simulink model "controle_manual_tuned_PID"  (Simulink 8.3)
settings: Solver=ode3  StartTime=0.0  StopTime=20  FixedStep=0.01  MaxStep=0.1  RelTol=1e-3
InitFcn:
  | % load parameters of the default quadrotor
  | disp('Quadrotor parameters loaded by InitFcn')
  | mdl_quadrotor
  | 
  | P_x=0.1;
  | I_x=0.001;
  | D_x=2;
  | 
  | P_y=0.1;
  | I_y=0.001;
  | D_y=2;
  | 
  | P_z=40;
  | I_z=0.01;
  | D_z=2;
undefined symbols (not defined in the file or in its folder): quad, sigbuilder_block
libraries: simulink x1
settings Model: Creator=corkep  LastModifiedBy=kleber
settings OptimizationCC: ExpressionDepthLimit=2147483647
settings DebuggingCC: FcnCallInpInsideContextMsg=UseLocalSettings  FrameProcessingCompatibilityMsg=error

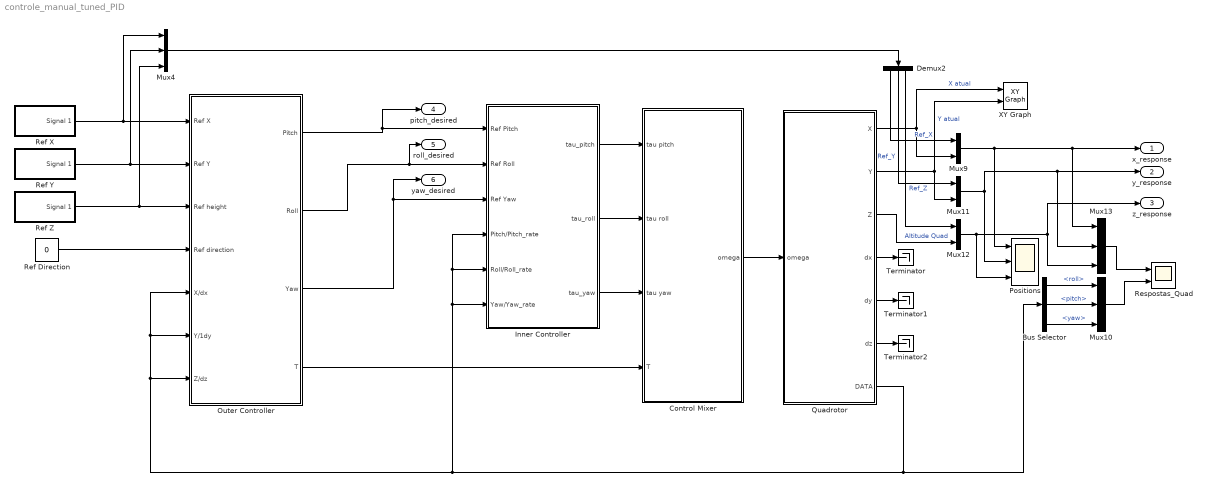
== system controle_manual_tuned_PID ==
  Bus Selector : BusSelector  OutputSignals=roll,pitch,yaw
  Control Mixer : Subsystem  AncestorBlock=roblocks/Dynamics/Control Mixer 4
      mask help: Quadrotor control mixer
      mask Help:
      | Determine rotor speeds based on desired torques and thrust.
      | 
      | <b>Inputs::</b>
      | 
      | tau pitch (1x1)  desired pitching torque [Nm]
      | tau roll (1x1)   desired rolling torque [Nm]
      | tau yaw (1x1)    desired yawing torque [Nm]
      | T (1x1)          desired thrust [N]
      | 
      | <b>Outputs::</b>
      | 
      | w1 (1x1) angular velocity of rotor 1 [rad]
      | w2 (1x1) angular velocity of rotor 2 [rad]
      | w3 (1x1) angular velocity of rotor 3 [rad]
      | w4 (1x1) angular velocity of rotor 4 [rad]
      | 
      | <b>Notes::</b>
      | 
      | - Assumes the rotor labelling convention of RVC Fig 4.16.
      | - The quadrotor is underactuated and has only 4 inputs.
  Demux2 : Demux  Outputs=3
  Inner Controller : Subsystem
  Mux10 : Mux  Inputs=3
  Mux11 : Mux  Inputs=2
  Mux12 : Mux  Inputs=2
  Mux13 : Mux  Inputs=3
  Mux4 : Mux  Inputs=3
  Mux9 : Mux  Inputs=2
  Outer Controller : Subsystem
  Positions : Scope  NumInputPorts=3
      settings: ShowLegends=on  YMin=-0.1~-0.05~0  YMax=1.1~0.5~1.1  SaveName=ScopeData4
  Quadrotor : Subsystem  AncestorBlock=roblocks/Dynamics/Quadrotor  mask{quad=quad}
      mask prompts: quad "Quadrotor params"
      mask help: Quadrotor dynamics
      mask Help:
      | Integrate spatial velocity to update pose represented as a homogeneous
      | transformation.
      | 
      | <b>Parameters::</b>
      | 
      | q (struct)  A structure containing quadrotor dynamics
      | 
      | The elements of q are:
      | 
      |  J         Flyer rotational inertia matrix (3x3)
      |  h         Height of rotors above CoG (1x1)
      |  d         Length of flyer arms (1x1)
      |  nb        Number of blades per rotor (1x1)
      |  r         Rotor radius (1x1)
      |  c         Blade chord (1x1)
      |  e         Flapping hinge offset (1x1)
      |  Mb        Rotor blade mass (1x1)
      |  Mc        Estimated hub clamp mass (1x1)
      |  ec        Blade root clamp displacement (1x1)
      |  Ib        Rotor blade rotational inertia (1x1)
      |  Ic        Estimated root clamp inertia (1x1)
      |  mb        Static blade moment (1x1)
      |  Ir        Total rotor inertia (1x1)
      |  Ct        Non-dim. thrust coefficient (1x1)
      |  Cq        Non-dim. torque coefficient (1x1)
      |  sigma     Rotor solidity ratio (1x1)
      |  thetat    Blade tip angle (1x1)
      |  theta0    Blade root angle (1x1)
      |  theta1    Blade twist angle (1x1)
      |  theta75   3/4 blade angle (1x1)
      |  thetai    Blade ideal root approximation (1x1)
      |  a         Lift slope gradient (1x1)
      |  A         Rotor disc area (1x1)
      |  gamma     Lock number (1x1)
      | 
      | 
      | <b>Inputs::</b>
      | 
      | w1 (1x1) angular velocity of rotor 1 [rad]
      | w2 (1x1) angular velocity of rotor 2 [rad]
      | w3 (1x1) angular velocity of rotor 3 [rad]
      | w4 (1x1) angular velocity of rotor 4 [rad]
      | 
      | <b>Outputs::</b>
      | 
      | X (1x12) state vector (x, y, z, thr, thp, thy, xd, yd, zd, thrd, thpd, thyd)
      | 
      | (x,y,z) is the position in the world frame [m]
      | (thr, thp, thy) the roll/pitch/yaw orientation in the world frame [rad]
      | (xd,yd,zd) is the velocity in the body frame [m]
      | (thrd,thpd,thyd) is the roll/pitch/yaw rates in the body frame [rad/s]
      | 
      | <b>Notes::</b>
      | 
      | - See also mdl_quadrotor which defines parameters for the ANU X4 flyer.
  Ref Direction : Constant  Value=0  SampleTime=0
  Ref X : Subsystem  Tag=STV Subsys  LoadFcn=sigbuilder_block('load');  StartFcn=sigbuilder_block('start');  StopFcn=sigbuilder_block('stop');  ClipboardFcn=sigbuilder_block('clipboard');  mask(Sigbuilder block){}
      mask help: Sigbuilder GUI
      mask init:
      | if ~strcmp(get_param(bdroot(gcbh),'SimulationStatus'),'stopped') tuvar = sigbuilder_block('maskInit'); end
      settings: CopyFcn=sigbuilder_block('copy');  DeleteFcn=sigbuilder_block('delete');  ModelCloseFcn=sigbuilder_block('modelClose');  PreSaveFcn=sigbuilder_block('preSave');  PauseFcn=sigbuilder_block('pause')  ContinueFcn=sigbuilder_block('continue')  NameChangeFcn=sigbuilder_block('namechange');  OpenFcn=sigbuilder_block('open',[73.6 132.8 512 286.4 ]);  CloseFcn=sigbuilder_block('close');
      mask Display: plot(0,0,100,100,[10,10,40,40,10],[80,20,20,80,80],[40,10],[50,50], [40,27,10],[65,72,56],[40,25,25,10],[28,28,43,43]);
  Ref Y : Subsystem  Tag=STV Subsys  LoadFcn=sigbuilder_block('load');  StartFcn=sigbuilder_block('start');  StopFcn=sigbuilder_block('stop');  ClipboardFcn=sigbuilder_block('clipboard');  mask(Sigbuilder block){}
      mask help: Sigbuilder GUI
      mask init:
      | if ~strcmp(get_param(bdroot(gcbh),'SimulationStatus'),'stopped') tuvar = sigbuilder_block('maskInit'); end
      settings: CopyFcn=sigbuilder_block('copy');  DeleteFcn=sigbuilder_block('delete');  ModelCloseFcn=sigbuilder_block('modelClose');  PreSaveFcn=sigbuilder_block('preSave');  PauseFcn=sigbuilder_block('pause')  ContinueFcn=sigbuilder_block('continue')  NameChangeFcn=sigbuilder_block('namechange');  OpenFcn=sigbuilder_block('open',[50.4 76.8 509.6 480.8 ]);  CloseFcn=sigbuilder_block('close');
      mask Display: plot(0,0,100,100,[10,10,40,40,10],[80,20,20,80,80],[40,10],[50,50], [40,27,10],[65,72,56],[40,25,25,10],[28,28,43,43]);
  Ref Z : Subsystem  Tag=STV Subsys  LoadFcn=sigbuilder_block('load');  StartFcn=sigbuilder_block('start');  StopFcn=sigbuilder_block('stop');  ClipboardFcn=sigbuilder_block('clipboard');  mask(Sigbuilder block){}
      mask help: Sigbuilder GUI
      mask init:
      | if ~strcmp(get_param(bdroot(gcbh),'SimulationStatus'),'stopped') tuvar = sigbuilder_block('maskInit'); end
      settings: CopyFcn=sigbuilder_block('copy');  DeleteFcn=sigbuilder_block('delete');  ModelCloseFcn=sigbuilder_block('modelClose');  PreSaveFcn=sigbuilder_block('preSave');  PauseFcn=sigbuilder_block('pause')  ContinueFcn=sigbuilder_block('continue')  NameChangeFcn=sigbuilder_block('namechange');  OpenFcn=sigbuilder_block('open',[566.4 -21.6 526.4 528.8 ]);  CloseFcn=sigbuilder_block('close');
      mask Display: plot(0,0,100,100,[10,10,40,40,10],[80,20,20,80,80],[40,10],[50,50], [40,27,10],[65,72,56],[40,25,25,10],[28,28,43,43]);
  Respostas_Quad : Scope  NumInputPorts=2
      settings: ShowLegends=on  YMin=-8~-0.0005  YMax=1~0.0105  SaveName=ScopeData5
  Terminator : Terminator
  Terminator1 : Terminator
  Terminator2 : Terminator
  XY Graph : simulink/Sinks/XY Graph  xmin=0  xmax=3  ymin=0  ymax=3  st=-1
  x_response : Outport
  y_response : Outport  Port=2
  z_response : Outport  Port=3
  pitch_desired : Outport  Port=4
  roll_desired : Outport  Port=5
  yaw_desired : Outport  Port=6
  wires:
  Outer Controller/4(T) -> Control Mixer/4(T)
  Control Mixer/1(omega) -> Quadrotor/1(omega)
  Inner Controller/1(tau_pitch) -> Control Mixer/1(tau pitch)
  Inner Controller/2(tau_roll) -> Control Mixer/2(tau roll)
  Inner Controller/3(tau_yaw) -> Control Mixer/3(tau yaw)
  Ref X/1(Signal 1) -> Mux4/1, Outer Controller/1(Ref X)
  Ref Z/1(Signal 1) -> Outer Controller/3(Ref height), Mux4/3
  Ref Direction/1 -> Outer Controller/4(Ref direction)
  Outer Controller/3(Yaw) -> yaw_desired/1, Inner Controller/3(Ref Yaw)
  Ref Y/1(Signal 1) -> Mux4/2, Outer Controller/2(Ref Y)
  Mux4/1 -> Demux2/1
  Quadrotor/7(DATA) -> Bus Selector/1, Inner Controller/6(Yaw/Yaw_rate), Inner Controller/5(Roll/Roll_rate), Inner Controller/4(Pitch/Pitch_rate), Outer Controller/5(X/dx), Outer Controller/6(Y/1dy), Outer Controller/7(Z/dz)
  Mux9/1 -> Mux13/1, x_response/1, Positions/1
  Mux12/1 -> Mux13/3, z_response/1, Positions/3
  Mux11/1 -> Positions/2, Mux13/2, y_response/1
  Mux13/1 -> Respostas_Quad/1
  Mux10/1 -> Respostas_Quad/2
  Bus Selector/2 -> Mux10/2  "<pitch>"
  Bus Selector/1 -> Mux10/1  "<roll>"
  Quadrotor/1(X) -> XY Graph/1, Mux9/2  "X atual"
  Quadrotor/3(Z) -> Mux12/2  "Altitude Quad"
  Bus Selector/3 -> Mux10/3  "<yaw>"
  Quadrotor/2(Y) -> Mux11/2, XY Graph/2  "Y atual"
  Demux2/1 -> Mux9/1  "Ref_X"
  Demux2/2 -> Mux11/1  "Ref_Y"
  Demux2/3 -> Mux12/1  "Ref_Z"
  Quadrotor/4(dx) -> Terminator/1
  Quadrotor/5(dy) -> Terminator1/1
  Quadrotor/6(dz) -> Terminator2/1
  Outer Controller/1(Pitch) -> pitch_desired/1, Inner Controller/1(Ref Pitch)
  Outer Controller/2(Roll) -> roll_desired/1, Inner Controller/2(Ref Roll)

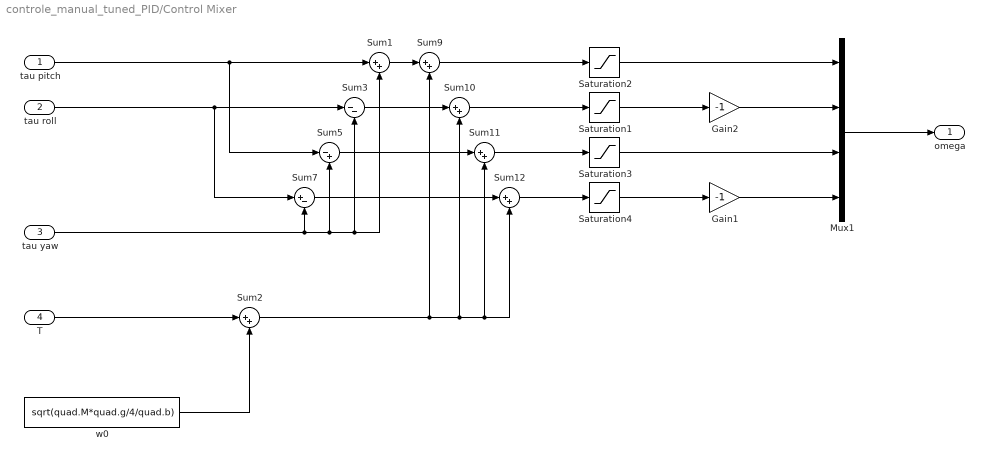
== system controle_manual_tuned_PID/Control Mixer ==
  tau pitch : Inport
  tau roll : Inport  Port=2
  tau yaw : Inport  Port=3
  T : Inport  Port=4
  Gain1 : Gain  Gain=-1
  Gain2 : Gain  Gain=-1
  Mux1 : Mux
  Saturation{1..4} (4 alike) : Saturate  UpperLimit=1000  LowerLimit=700
  Sum{1..2,9..12} (6 alike) : Sum  Inputs=|++  SaturateOnIntegerOverflow=on  InputSameDT=on  OutDataTypeStr=Inherit: Same as first input
  Sum3 : Sum  Inputs=|--  SaturateOnIntegerOverflow=on  InputSameDT=on  OutDataTypeStr=Inherit: Same as first input
  Sum5 : Sum  Inputs=|-+  SaturateOnIntegerOverflow=on  InputSameDT=on  OutDataTypeStr=Inherit: Same as first input
  Sum7 : Sum  Inputs=|+-  SaturateOnIntegerOverflow=on  InputSameDT=on  OutDataTypeStr=Inherit: Same as first input
  w0 : Constant  Value=sqrt(quad.M*quad.g/4/quad.b)  SampleTime=0
  omega : Outport
  wires:
  Mux1/1 -> omega/1
  Gain2/1 -> Mux1/2
  tau yaw/1 -> Sum7/2, Sum5/2, Sum3/2, Sum1/2
  Saturation2/1 -> Mux1/1
  Saturation1/1 -> Gain2/1
  Saturation3/1 -> Mux1/3
  Saturation4/1 -> Gain1/1
  tau pitch/1 -> Sum5/1, Sum1/1
  Sum1/1 -> Sum9/1
  Sum3/1 -> Sum10/1
  Sum5/1 -> Sum11/1
  Sum7/1 -> Sum12/1
  Sum9/1 -> Saturation2/1
  Sum10/1 -> Saturation1/1
  Sum11/1 -> Saturation3/1
  Sum12/1 -> Saturation4/1
  tau roll/1 -> Sum7/1, Sum3/1
  Gain1/1 -> Mux1/4
  Sum2/1 -> Sum9/2, Sum11/2, Sum12/2, Sum10/2
  T/1 -> Sum2/1
  w0/1 -> Sum2/2

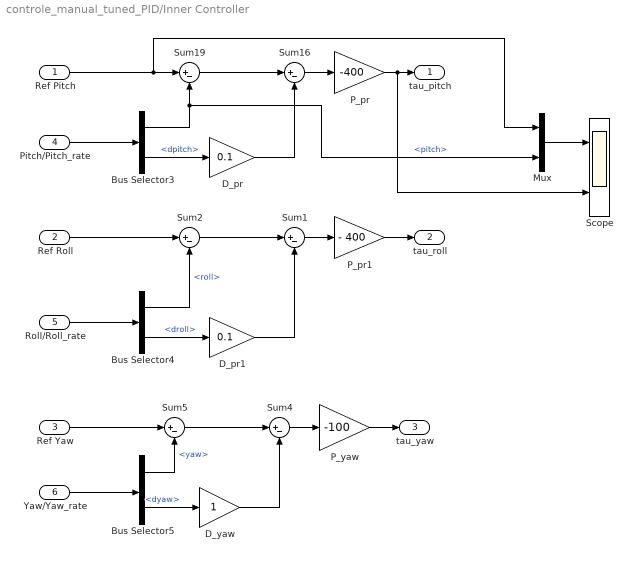
== system controle_manual_tuned_PID/Inner Controller ==
  Ref Pitch : Inport
  Ref Roll : Inport  Port=2
  Ref Yaw : Inport  Port=3
  Pitch/Pitch_rate : Inport  Port=4
  Roll/Roll_rate : Inport  Port=5
  Yaw/Yaw_rate : Inport  Port=6
  Bus Selector3 : BusSelector  OutputSignals=pitch,dpitch
  Bus Selector4 : BusSelector  OutputSignals=roll,droll
  Bus Selector5 : BusSelector  OutputSignals=yaw,dyaw
  D_pr : Gain  Gain=0.1
  D_pr1 : Gain  Gain=0.1
  D_yaw : Gain
  Mux : Mux  Inputs=2
  P_pr : Gain  Gain=-400
  P_pr1 : Gain  Gain=- 400
  P_yaw : Gain  Gain=-100
  Scope : Scope  NumInputPorts=2
      settings: YMin=-5~-5  YMax=5~5  SaveName=ScopeData3
  Sum{1..2,4..5,16,19} (6 alike) : Sum  Inputs=|+-
  tau_pitch : Outport
  tau_roll : Outport  Port=2
  tau_yaw : Outport  Port=3
  wires:
  Sum19/1 -> Sum16/1
  Sum16/1 -> P_pr/1
  P_pr/1 -> Scope/2, tau_pitch/1
  D_pr/1 -> Sum16/2
  Bus Selector3/2 -> D_pr/1  "<dpitch>"
  Bus Selector3/1 -> Mux/2, Sum19/2  "<pitch>"
  Sum2/1 -> Sum1/1
  Sum1/1 -> P_pr1/1
  P_pr1/1 -> tau_roll/1
  D_pr1/1 -> Sum1/2
  Bus Selector4/2 -> D_pr1/1  "<droll>"
  Ref Pitch/1 -> Mux/1, Sum19/1
  Pitch/Pitch_rate/1 -> Bus Selector3/1
  Roll/Roll_rate/1 -> Bus Selector4/1
  Bus Selector4/1 -> Sum2/2  "<roll>"
  Ref Roll/1 -> Sum2/1
  Bus Selector5/1 -> Sum5/2  "<yaw>"
  Sum4/1 -> P_yaw/1
  Bus Selector5/2 -> D_yaw/1  "<dyaw>"
  D_yaw/1 -> Sum4/2
  Sum5/1 -> Sum4/1
  P_yaw/1 -> tau_yaw/1
  Yaw/Yaw_rate/1 -> Bus Selector5/1
  Ref Yaw/1 -> Sum5/1
  Mux/1 -> Scope/1

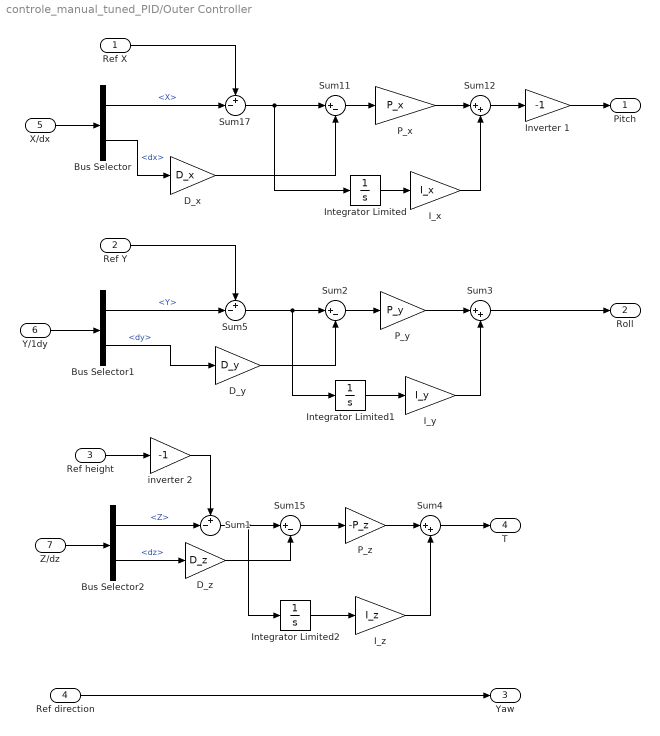
== system controle_manual_tuned_PID/Outer Controller ==
  Ref X : Inport
  Ref Y : Inport  Port=2
  Ref height : Inport  Port=3
  Ref direction : Inport  Port=4
  X/dx : Inport  Port=5
  Y/1dy : Inport  Port=6
  Z/dz : Inport  Port=7
  Bus Selector : BusSelector  OutputSignals=X,dx
  Bus Selector1 : BusSelector  OutputSignals=Y,dy
  Bus Selector2 : BusSelector  OutputSignals=Z,dz
  D_x : Gain  Gain=D_x
  D_y : Gain  Gain=D_y
  D_z : Gain  Gain=D_z
  I_x : Gain  Gain=I_x
  I_y : Gain  Gain=I_y
  I_z : Gain  Gain=I_z
  Integrator Limited : Integrator  LimitOutput=on  UpperSaturationLimit=1  LowerSaturationLimit=0
  Integrator Limited1 : Integrator  LimitOutput=on  UpperSaturationLimit=1  LowerSaturationLimit=0
  Integrator Limited2 : Integrator  LimitOutput=on  UpperSaturationLimit=1  LowerSaturationLimit=0
  Inverter 1 : Gain  Gain=-1
  P_x : Gain  Gain=P_x
  P_y : Gain  Gain=P_y
  P_z : Gain  Gain=-P_z
  Sum1 : Sum  Inputs=+-|
  Sum11 : Sum  Inputs=|+-
  Sum12 : Sum  Inputs=|++
  Sum15 : Sum  Inputs=|+-
  Sum17 : Sum  Inputs=+-|
  Sum2 : Sum  Inputs=|+-
  Sum3 : Sum  Inputs=|++
  Sum4 : Sum  Inputs=|++
  Sum5 : Sum  Inputs=+-|
  inverter 2 : Gain  Gain=-1
  Pitch : Outport
  Roll : Outport  Port=2
  Yaw : Outport  Port=3
  T : Outport  Port=4
  wires:
  Sum15/1 -> P_z/1
  Sum1/1 -> Sum15/1, Integrator Limited2/1
  Ref height/1 -> inverter 2/1
  Z/dz/1 -> Bus Selector2/1
  Ref X/1 -> Sum17/1
  Ref direction/1 -> Yaw/1
  Y/1dy/1 -> Bus Selector1/1
  inverter 2/1 -> Sum1/1
  Bus Selector2/1 -> Sum1/2  "<Z>"
  Bus Selector2/2 -> D_z/1  "<dz>"
  D_z/1 -> Sum15/2
  X/dx/1 -> Bus Selector/1
  Integrator Limited/1 -> I_x/1
  Bus Selector/1 -> Sum17/2  "<X>"
  P_x/1 -> Sum12/1
  Sum17/1 -> Sum11/1, Integrator Limited/1
  D_x/1 -> Sum11/2
  Sum11/1 -> P_x/1
  Bus Selector/2 -> D_x/1  "<dx>"
  I_x/1 -> Sum12/2
  Integrator Limited1/1 -> I_y/1
  Bus Selector1/1 -> Sum5/2  "<Y>"
  P_y/1 -> Sum3/1
  Sum5/1 -> Sum2/1, Integrator Limited1/1
  D_y/1 -> Sum2/2
  Sum2/1 -> P_y/1
  Bus Selector1/2 -> D_y/1  "<dy>"
  I_y/1 -> Sum3/2
  Sum12/1 -> Inverter 1/1
  Inverter 1/1 -> Pitch/1
  Sum3/1 -> Roll/1
  P_z/1 -> Sum4/1
  Sum4/1 -> T/1
  I_z/1 -> Sum4/2
  Integrator Limited2/1 -> I_z/1
  Ref Y/1 -> Sum5/1

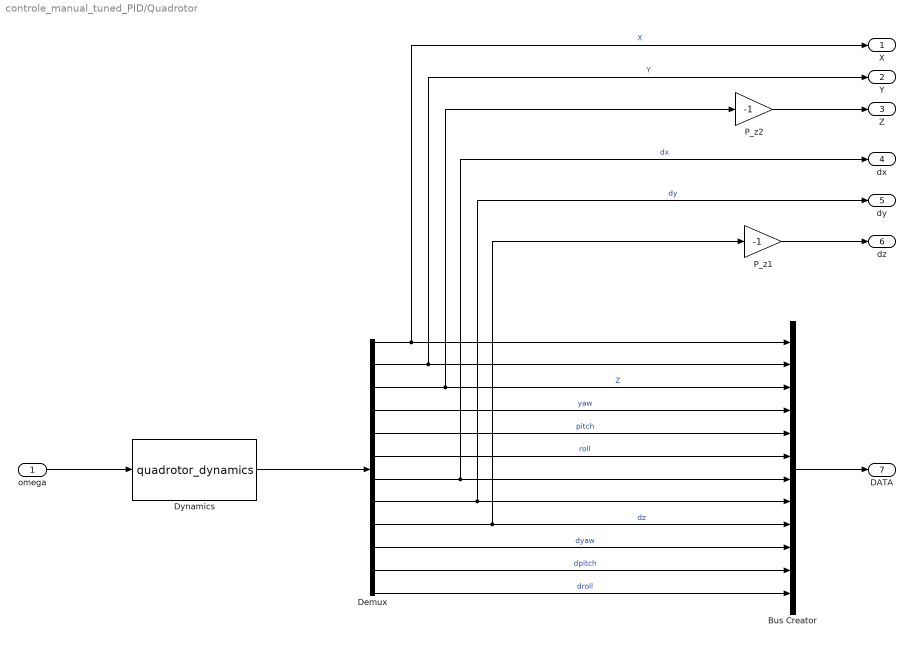
== system controle_manual_tuned_PID/Quadrotor ==
  omega : Inport
  Bus Creator : BusCreator  Inputs='X','Y','Z','yaw','pitch','roll','dx','dy','dz','dyaw','dpitch','droll'
  Demux : Demux  Outputs=12
  Dynamics : S-Function  FunctionName=quadrotor_dynamics  Parameters=quad  EnableBusSupport=off
  P_z1 : Gain  Gain=-1
  P_z2 : Gain  Gain=-1
  X : Outport
  Y : Outport  Port=2
  Z : Outport  Port=3
  dx : Outport  Port=4
  dy : Outport  Port=5
  dz : Outport  Port=6
  DATA : Outport  Port=7
  wires:
  Demux/1 -> X/1, Bus Creator/1  "X"
  Demux/3 -> Bus Creator/3, P_z2/1  "Z"
  Demux/4 -> Bus Creator/4  "yaw"
  Demux/5 -> Bus Creator/5  "pitch"
  omega/1 -> Dynamics/1
  Demux/7 -> dx/1, Bus Creator/7  "dx"
  Demux/9 -> P_z1/1, Bus Creator/9  "dz"
  Demux/2 -> Y/1, Bus Creator/2  "Y"
  Demux/6 -> Bus Creator/6  "roll"
  Demux/8 -> dy/1, Bus Creator/8  "dy"
  Bus Creator/1 -> DATA/1
  Dynamics/1 -> Demux/1
  Demux/10 -> Bus Creator/10  "dyaw"
  Demux/11 -> Bus Creator/11  "dpitch"
  Demux/12 -> Bus Creator/12  "droll"
  P_z2/1 -> Z/1
  P_z1/1 -> dz/1

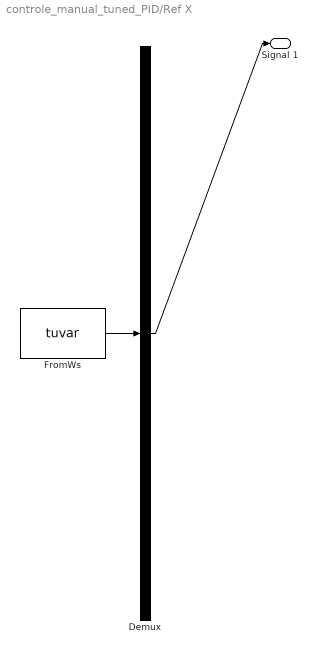
== system controle_manual_tuned_PID/Ref X ==
  Demux : Demux  Tag=STV Demux  Outputs=1
  FromWs : FromWorkspace  Tag=STV FromWs  VariableName=tuvar  SampleTime=0  SigBuilderData=DataTag0  VnvData=DataTag1
      SigBuilderData=|
      | common.afterFinalStr = 'Extrapolate'
      | common.sampleTime = 0
      | dataSet.timeRange = [0 130]
      | dataSet.name = 'Group 1'
      | sbobj.Name = 'Signal Builder'
      | sbobj.Groups.Name = 'Group 1'
      | sbobj.Groups.Signals.Name = 'Signal 1'
      | sbobj.Groups.Signals.XData = [0 5 7 15 60 65 130]
      | sbobj.Groups.Signals.YData = [0 0 1 1 1 1.5 1.5]
      | sbobj.Groups.TimeRange = [0 130]
  Signal 1 : Outport  Tag=STV Outport
  wires:
  FromWs/1 -> Demux/1
  Demux/1 -> Signal 1/1

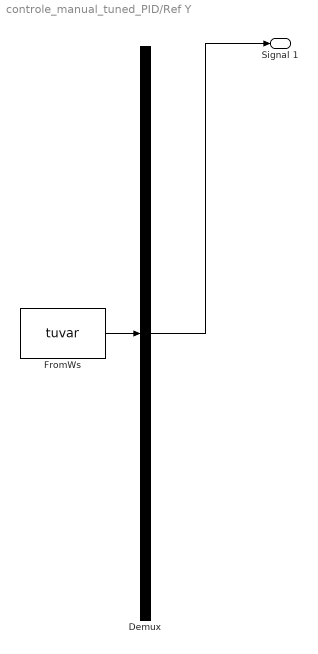
== system controle_manual_tuned_PID/Ref Y ==
  Demux : Demux  Tag=STV Demux  Outputs=1
  FromWs : FromWorkspace  Tag=STV FromWs  VariableName=tuvar  SampleTime=0  SigBuilderData=DataTag2  VnvData=DataTag3
      SigBuilderData=|
      | common.afterFinalStr = 'Extrapolate'
      | common.sampleTime = 0
      | dataSet.timeRange = [0 130]
      | dataSet.name = 'Group 1'
      | sbobj.Name = 'Signal Builder'
      | sbobj.Groups.Name = 'Group 1'
      | sbobj.Groups.Signals.Name = 'Signal 1'
      | sbobj.Groups.Signals.XData = [0 5 10 30 35 60 65 90 95 130]
      | sbobj.Groups.Signals.YData = [0 0 0.5 0.5 2.5 2.5 0.5 0.5 2.5 2.5]
      | sbobj.Groups.TimeRange = [0 130]
  Signal 1 : Outport  Tag=STV Outport
  wires:
  Demux/1 -> Signal 1/1
  FromWs/1 -> Demux/1

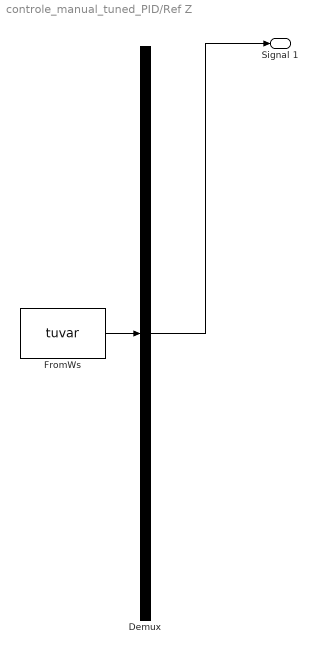
== system controle_manual_tuned_PID/Ref Z ==
  Demux : Demux  Tag=STV Demux  Outputs=1
  FromWs : FromWorkspace  Tag=STV FromWs  VariableName=tuvar  SampleTime=0  SigBuilderData=DataTag4  VnvData=DataTag5
      SigBuilderData=|
      | common.afterFinalStr = 'Extrapolate'
      | common.sampleTime = 0
      | dataSet.timeRange = [0 130]
      | dataSet.name = 'Group 1'
      | sbobj.Name = 'Signal Builder'
      | sbobj.Groups.Name = 'Group 1'
      | sbobj.Groups.Signals.Name = 'Signal 1'
      | sbobj.Groups.Signals.XData = [0 5 15 20 25 30 45 50 55 60 75 80 85 90 105 110 115 120 130]
      | sbobj.Groups.Signals.YData = [0 1 1 0.2 0.2 1 1 0.2 0.2 1 1 0.2 0.2 1 1 0.2 0.2 1 1]
      | sbobj.Groups.TimeRange = [0 130]
  Signal 1 : Outport  Tag=STV Outport
  wires:
  Demux/1 -> Signal 1/1
  FromWs/1 -> Demux/1
